simulink model "Reference"  (R2015a)
settings: Solver=ode45  StartTime=0.0  StopTime=5  RelTol=1e-3
model workspace (MAT data in the model file):
  a_0 = 1
  a_1 = 1.25
  a_2 = 0.5
  a_3 = 0.025
  s_1 = 0.1
  s_2 = 0.2
  s_3 = 0.3
settings Model: Creator=ry0  LastModifiedBy=ry0

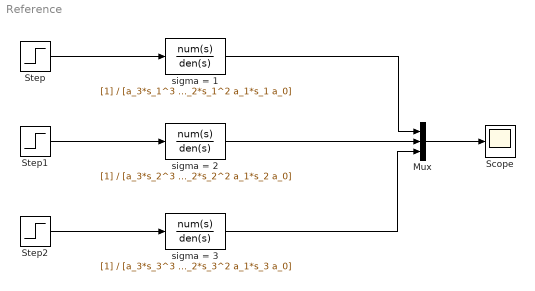
== system Reference ==
  Mux : Mux  Inputs=3
  Scope : Scope
      settings: TimeRange=30  YMin=0  YMax=500
  Step : Step  Time=0  SampleTime=0
  Step1 : Step  Time=0  SampleTime=0
  Step2 : Step  Time=0  SampleTime=0
  sigma = 1 : TransferFcn  Denominator=[a_3*s_1^3 a_2*s_1^2 a_1*s_1 a_0]
  sigma = 2 : TransferFcn  Denominator=[a_3*s_2^3 a_2*s_2^2 a_1*s_2 a_0]
  sigma = 3 : TransferFcn  Denominator=[a_3*s_3^3 a_2*s_3^2 a_1*s_3 a_0]
  wires:
  Mux/1 -> Scope/1
  sigma = 1/1 -> Mux/1
  sigma = 2/1 -> Mux/2
  sigma = 3/1 -> Mux/3
  Step/1 -> sigma = 1/1
  Step1/1 -> sigma = 2/1
  Step2/1 -> sigma = 3/1
